simulink model "DIK_mdl"  (R2013a)
settings: Solver=ode45  StartTime=0.0  StopTime=10.0  RelTol=1e-3
undefined symbols (not defined in the file or in its folder): Conv_loop, ToSimulink_Y_Signals2VRML, Y_J_DIK
libraries: simulink x6, vrlib x1
settings Model: Creator=root  LastModifiedBy=root

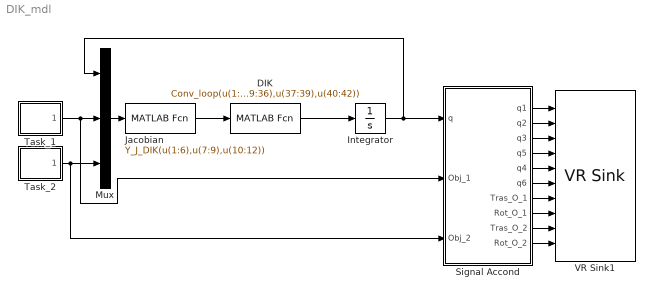
== system DIK_mdl ==
  DIK : MATLABFcn  MATLABFcn=Conv_loop(u(1:18),u(19:36),u(37:39),u(40:42))  OutputDimensions=6
  Integrator : Integrator
  Jacobian : MATLABFcn  MATLABFcn=Y_J_DIK(u(1:6),u(7:9),u(10:12))  OutputDimensions=42
  Mux : Mux  Inputs=3
  Signal Accond : Subsystem
  Task_1 : Subsystem
  Task_2 : Subsystem
  VR Sink1 : vrlib/VR Sink  InstantiateOnLoad=on  SampleTime=0.1  ViewEnable=on  RemoteChange=off  RemoteView=off  FieldsWritten=Q_1.rotation.4.1.1.double#Q_2.rotation.4.1.1.double#Q_3_Der.rotation.4.1.1.double#Q_5.rotation.4.1.1.double#Q_4_Izq.rotation.4.1.1.double#Q_6.rotation.4.1.1.double#Tras_Objective1.translation.3.1.1.double#RY_Obj1.rotation.4.1.1.double#Tras_Objective2.translation.3.1.1.double#RY_Obj2.rotation.4.1.1.double  WorldFileName=Y.WRL  AutoView=off  VideoDimensions=[]  AllowVariableSize=off
  wires:
  Jacobian/1 -> DIK/1
  DIK/1 -> Integrator/1
  Mux/1 -> Jacobian/1
  Integrator/1 -> Signal Accond/1(q), Mux/1
  Task_1/1(Task 1) -> Signal Accond/2(Obj_1), Mux/2
  Task_2/1(Task 2) -> Mux/3, Signal Accond/3(Obj_2)
  Signal Accond/1(q1) -> VR Sink1/1
  Signal Accond/10(Rot_O_2) -> VR Sink1/10
  Signal Accond/2(q2) -> VR Sink1/2
  Signal Accond/3(q3) -> VR Sink1/3
  Signal Accond/7(Tras_O_1) -> VR Sink1/7
  Signal Accond/4(q5) -> VR Sink1/4
  Signal Accond/5(q4) -> VR Sink1/5
  Signal Accond/9(Tras_O_2) -> VR Sink1/9
  Signal Accond/8(Rot_O_1) -> VR Sink1/8
  Signal Accond/6(q6) -> VR Sink1/6

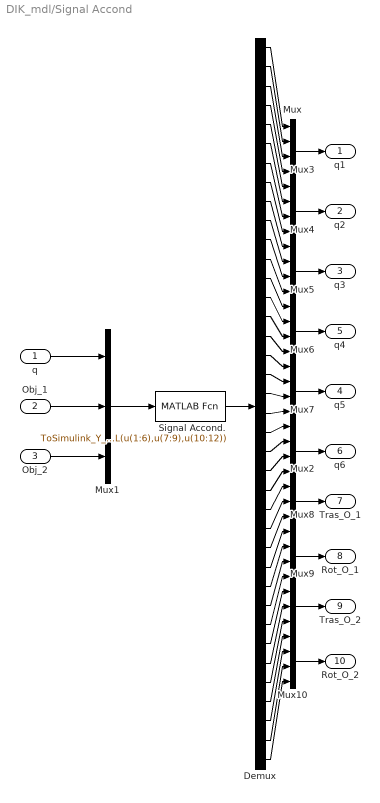
== system DIK_mdl/Signal Accond ==
  q : Inport
  Obj_1 : Inport  Port=2
  Obj_2 : Inport  Port=3
  Demux : Demux  Outputs=38
  Mux{,3..8,10} (8 alike) : Mux
  Mux1 : Mux  Inputs=3
  Mux2 : Mux  Inputs=3
  Mux9 : Mux  Inputs=3
  Signal Accond. : MATLABFcn  MATLABFcn=ToSimulink_Y_Signals2VRML(u(1:6),u(7:9),u(10:12))  OutputDimensions=38
  q1 : Outport
  q2 : Outport  Port=2
  q3 : Outport  Port=3
  q5 : Outport  Port=4
  q4 : Outport  Port=5
  q6 : Outport  Port=6
  Tras_O_1 : Outport  Port=7
  Rot_O_1 : Outport  Port=8
  Tras_O_2 : Outport  Port=9
  Rot_O_2 : Outport  Port=10
  wires:
  Signal Accond./1 -> Demux/1
  Mux1/1 -> Signal Accond./1
  Obj_1/1 -> Mux1/2
  Obj_2/1 -> Mux1/3
  q/1 -> Mux1/1
  Demux/33 -> Mux9/2
  Demux/7 -> Mux3/3
  Demux/20 -> Mux6/4
  Demux/6 -> Mux3/2
  Demux/3 -> Mux/3
  Demux/27 -> Mux2/3
  Demux/28 -> Mux8/1
  Demux/29 -> Mux8/2
  Demux/34 -> Mux9/3
  Demux/35 -> Mux10/1
  Demux/36 -> Mux10/2
  Demux/19 -> Mux6/3
  Demux/37 -> Mux10/3
  Demux/10 -> Mux4/2
  Demux/18 -> Mux6/2
  Demux/1 -> Mux/1
  Demux/4 -> Mux/4
  Demux/16 -> Mux5/4
  Demux/5 -> Mux3/1
  Demux/30 -> Mux8/3
  Demux/31 -> Mux8/4
  Demux/32 -> Mux9/1
  Demux/15 -> Mux5/3
  Demux/2 -> Mux/2
  Demux/13 -> Mux5/1
  Demux/22 -> Mux7/2
  Demux/23 -> Mux7/3
  Demux/24 -> Mux7/4
  Demux/26 -> Mux2/2
  Demux/12 -> Mux4/4
  Demux/8 -> Mux3/4
  Demux/38 -> Mux10/4
  Demux/9 -> Mux4/1
  Demux/25 -> Mux2/1
  Demux/17 -> Mux6/1
  Demux/11 -> Mux4/3
  Demux/21 -> Mux7/1
  Demux/14 -> Mux5/2
  Mux/1 -> q1/1
  Mux3/1 -> q2/1
  Mux4/1 -> q3/1
  Mux5/1 -> q4/1
  Mux6/1 -> q5/1
  Mux7/1 -> q6/1
  Mux2/1 -> Tras_O_1/1
  Mux8/1 -> Rot_O_1/1
  Mux9/1 -> Tras_O_2/1
  Mux10/1 -> Rot_O_2/1

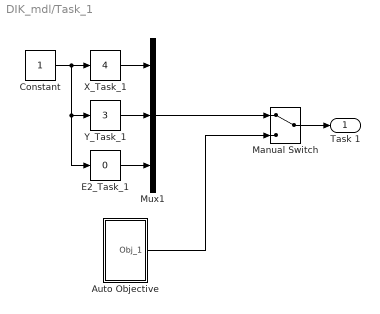
== system DIK_mdl/Task_1 ==
  Auto Objective : Subsystem
  Constant : Constant
  E2_Task_1 : simulink/Math Operations/Slider Gain  low=-6.28  gain=0  high=6.28
  Manual Switch : ManualSwitch
  Mux1 : Mux  Inputs=3
  X_Task_1 : simulink/Math Operations/Slider Gain  low=-5  gain=4  high=5
  Y_Task_1 : simulink/Math Operations/Slider Gain  low=-5  gain=3  high=5
  Task 1 : Outport
  wires:
  X_Task_1/1 -> Mux1/1
  Constant/1 -> X_Task_1/1, E2_Task_1/1, Y_Task_1/1
  E2_Task_1/1 -> Mux1/3
  Y_Task_1/1 -> Mux1/2
  Auto Objective/1(Obj_1) -> Manual Switch/2
  Mux1/1 -> Manual Switch/1
  Manual Switch/1 -> Task 1/1

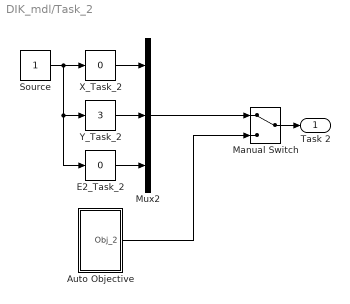
== system DIK_mdl/Task_2 ==
  Auto Objective : Subsystem
  E2_Task_2 : simulink/Math Operations/Slider Gain  low=-6.28  gain=0  high=6.28
  Manual Switch : ManualSwitch
  Mux2 : Mux  Inputs=3
  Source : Constant
  X_Task_2 : simulink/Math Operations/Slider Gain  low=-5  gain=0  high=5
  Y_Task_2 : simulink/Math Operations/Slider Gain  low=-5  gain=3  high=5
  Task 2 : Outport
  wires:
  Source/1 -> E2_Task_2/1, Y_Task_2/1, X_Task_2/1
  Y_Task_2/1 -> Mux2/2
  E2_Task_2/1 -> Mux2/3
  X_Task_2/1 -> Mux2/1
  Manual Switch/1 -> Task 2/1
  Mux2/1 -> Manual Switch/1
  Auto Objective/1(Obj_2) -> Manual Switch/2

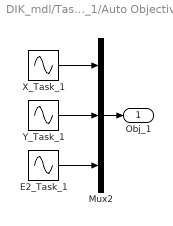
== system DIK_mdl/Task_1/Auto Objective ==
  E2_Task_1 : Sin  SineType=Sample based  Amplitude=6.28  SampleTime=.01
  Mux2 : Mux  Inputs=3
  X_Task_1 : Sin  SineType=Sample based  Amplitude=5  SampleTime=0.01
  Y_Task_1 : Sin  SineType=Sample based  Amplitude=5  SampleTime=0.01
  Obj_1 : Outport
  wires:
  Y_Task_1/1 -> Mux2/2
  X_Task_1/1 -> Mux2/1
  Mux2/1 -> Obj_1/1
  E2_Task_1/1 -> Mux2/3

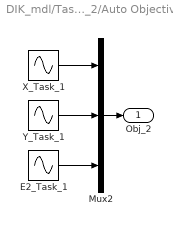
== system DIK_mdl/Task_2/Auto Objective ==
  E2_Task_1 : Sin  SineType=Sample based  Amplitude=6.28  SampleTime=.01
  Mux2 : Mux  Inputs=3
  X_Task_1 : Sin  SineType=Sample based  Amplitude=5  SampleTime=0.01
  Y_Task_1 : Sin  SineType=Sample based  Amplitude=5  SampleTime=0.01
  Obj_2 : Outport
  wires:
  Y_Task_1/1 -> Mux2/2
  X_Task_1/1 -> Mux2/1
  Mux2/1 -> Obj_2/1
  E2_Task_1/1 -> Mux2/3
